simulink model "Untitled1"  (Simulink 8.2)
settings: Solver=ode5  StartTime=0.0  StopTime=1415  FixedStep=0.5  RelTol=1e-3
settings Model: Creator=Satadru  LastModifiedBy=SD
settings DataIOCC: SaveOutput=off  SaveTime=off
settings DebuggingCC: FcnCallInpInsideContextMsg=EnableAllAsWarning
settings GRTTargetCC: CombineOutputUpdateFcns=on  GRTInterface=off

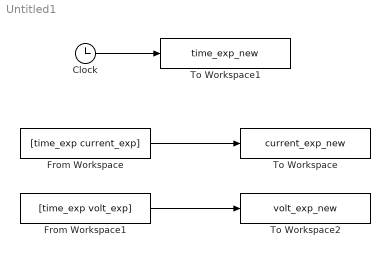
== system Untitled1 ==
  Clock : Clock
  From Workspace : FromWorkspace  VariableName=[time_exp current_exp]
  From Workspace1 : FromWorkspace  VariableName=[time_exp volt_exp]
  To Workspace : ToWorkspace  VariableName=current_exp_new  SampleTime=-1
  To Workspace1 : ToWorkspace  VariableName=time_exp_new  SampleTime=-1
  To Workspace2 : ToWorkspace  VariableName=volt_exp_new  SampleTime=-1
  wires:
  From Workspace/1 -> To Workspace/1
  Clock/1 -> To Workspace1/1
  From Workspace1/1 -> To Workspace2/1
